simulink model "cinematicabloque"  (R2024b)
settings: Solver=VariableStepAuto  StartTime=0.0  StopTime=100  RelTol=1e-3
settings Model: Creator=tomya  LastModifiedBy=tomya

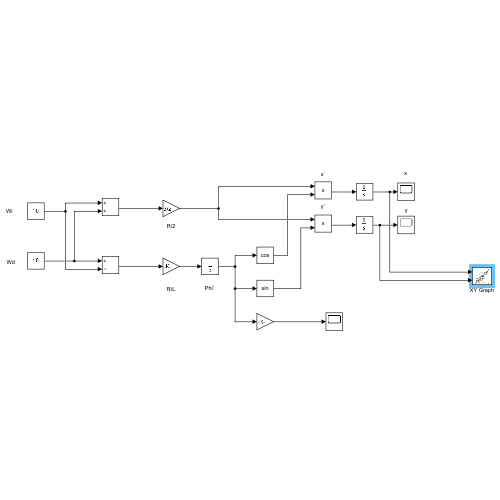
[thumbnail: Simulink's stored preview of the top-level diagram]
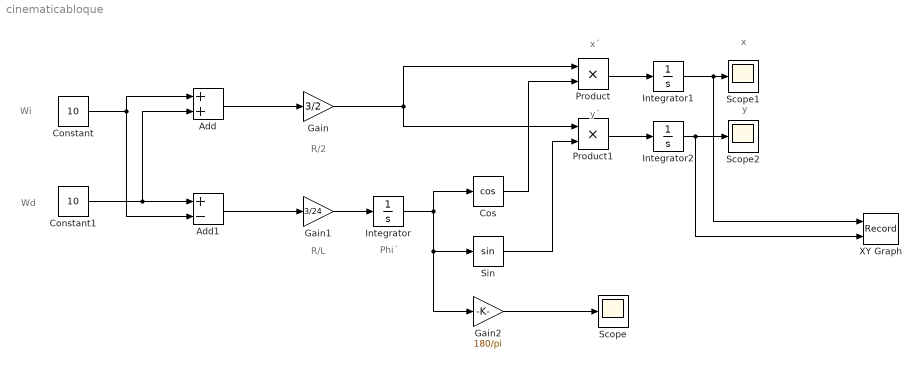
== system cinematicabloque ==
  note: y
  note: x
  note: Phi´
  note: y´
  note: x´
  note: R/L
  note: R/2
  note: Wd
  note: Wi
  Add : Sum
  Add1 : Sum  Inputs=+-
  Constant : Constant  Value=10
  Constant1 : Constant  Value=10
  Cos : Trigonometry  Operator=cos
  Gain : Gain  Gain=3/2
  Gain1 : Gain  Gain=3/24
  Gain2 : Gain  Gain=180/pi
  Integrator : Integrator
  Integrator1 : Integrator
  Integrator2 : Integrator
  Product : Product
  Product1 : Product
  Scope : Scope
  Scope1 : Scope
  Scope2 : Scope
  Sin : Trigonometry
  XY Graph : Record  FileSettingsInternal="{\"entries\":[{\"content\":{\"excelSettings\":{\"content\":{},\"type\":\"Streamout.ExcelSettings\"}},\"type\":\"Streamout.FileSettingStorage\",\"uuid\":\"\"}],\"packageUris\":[\"http:\\/\\/schema.mathworks.com\\/mf0\\/streamout_blocks\\/R2020a\"],\"version\":\"1.0\"}"  Layout=[1 1]  SignalsInternal="{\"entries\":[{\"content\":{\"signals\":[{\"content\":{\"blockPath\":[],\"dimensions\":[1],\"domain\":\"\",\"lineColor\":\"#a2142f\",\"plots\":[ 1 ],\"port\":1,\"sid\":[\"\"],\"signalID\":1,\"signalName\":\"Integrator1\"},\"type\":\"RecordBlkView.Signal\",\"uuid\":\"\"},{\"content\":{\"blockPath\":[],\"dimensions\":[1],\"domain\":\"\",\"lineColor\":\"#139fff\",\"plots\":[ 1 ],\"port\":2,\"sid\":[\"\"],\"signalID\":2,\"signalName\":\"Integrator2\"},\"type\":\"RecordBlkView.Signal\",\"uuid\":\"\"}]},\"type\":\"RecordBlkView.InputSignals\",\"uuid\":\"\"}],\"packageUris\":[\"http:\\/\\/schema.mathworks.com\\/mf0\\/streamout_blocks\\/R2020a\"],\"version\":\"1.0\"}"  VisualizationBindings="{\"xyplotplugin\":{\"info\":[{\"series\":[{\"bindingParametersList\":[{\"parameter\":\"X-Axis\",\"signalID\":1,\"signalName\":\"Integrator1\"},{\"parameter\":\"Y-Axis\",\"signalID\":2,\"signalName\":\"Integrator2\"}],\"seriesID\":0}],\"subplotID\":1}]}}"  CompatibilityTag=XY
  wires:
  Constant/1 -> Add1/2, Add/1
  Constant1/1 -> Add/2, Add1/1
  Add/1 -> Gain/1
  Add1/1 -> Gain1/1
  Gain1/1 -> Integrator/1
  Integrator/1 -> Cos/1, Sin/1, Gain2/1
  Gain/1 -> Product/1, Product1/1
  Cos/1 -> Product/2
  Sin/1 -> Product1/2
  Gain2/1 -> Scope/1
  Product/1 -> Integrator1/1
  Integrator1/1 -> XY Graph/1, Scope1/1
  Product1/1 -> Integrator2/1
  Integrator2/1 -> Scope2/1, XY Graph/2
